simulink model "PathPlanningSample"  (R2019b)
settings: Solver=VariableStepAuto  StartTime=0.0  StopTime=10.0  RelTol=1e-3
settings Model: Creator=Mouleeswar  LastModifiedBy=naika

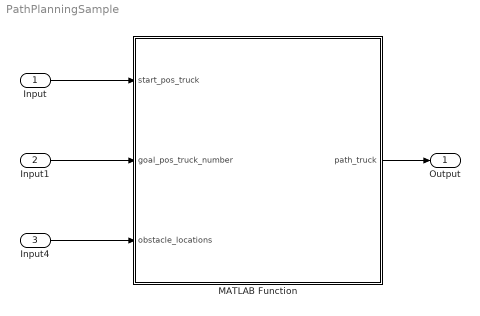
== system PathPlanningSample ==
  Input : Inport  OutDataTypeStr=double
  Input1 : Inport  Port=2  OutDataTypeStr=int16
  Input4 : Inport  Port=3  OutDataTypeStr=double
  MATLAB Function : MATLAB Function  TreatAsAtomicUnit=on
  Output : Outport  OutDataTypeStr=double
  wires:
  Input/1 -> MATLAB Function/1(start_pos_truck)
  Input1/1 -> MATLAB Function/2(goal_pos_truck_number)
  MATLAB Function/1(path_truck) -> Output/1
  Input4/1 -> MATLAB Function/3(obstacle_locations)

== matlab function PathPlanningSample/MATLAB Function ==
  data: start_pos_truck input; goal_pos_truck_number input; path_truck output; obstacle_locations input
function path_truck  = fcn(start_pos_truck, goal_pos_truck_number, obstacle_locations)
%% Input
S1 = start_pos_truck; %  [x-position y-position  angle  ]
E1 = goal_pos_truck_number; %  Dock number. Type:integer

obstacle = obstacle_locations; %Array containing the locations of all the obtacles. Example shown below.

%[ 5   6;
%  7   8;
% 100 500;
% 250 420;]

%% Output
%           [x-position y-position  angle   direction]
% units     [ meters      meters   radians      -    ]
% type      [ double      double    double   integer ]


% Ouput example
% path_truck1 = [100.01 100.02 1.56 1; % 
%                101.01 102.05 1.78 1;
%                101.01 102.05 1.78 -1;
%                101.01 102.05 1.78 -1];


    
edge = Map(obstacle);
costmap = vehicleCostmap(edge,'FreeThreshold',0.4);
 
vehicleDims = vehicleDimensions(98.5,19,'Wheelbase',62,'FrontOverhang',7.5,'RearOverhang',29);  % 4.5 m long, 1.7 m wide
NumCircles = 3;
ccConfig = inflationCollisionChecker(vehicleDims,'InflationRadius',5,'CenterPlacements',[0,0.5,1],'NumCircles',NumCircles);
costmap.CollisionChecker = ccConfig;

route = load('park_dock_points.mat')
routePlan = route.routePlan

dock_number = E1;
% park_number = 1;

% park = parking(park_number);
park = S1;
routePlan.StartPose(1,1) = park(1);
routePlan.StartPose(1,2) = park(2);
routePlan.StartPose(1,3) = park(3);


goal = docking(dock_number);
SP = HAS(goal,obstacle);

l=2;  % Number of wavepoints 

routePlan.EndPose(l,1) = SP(1);
routePlan.EndPose(l,2) = SP(2);
routePlan.EndPose(l,3) = SP(3);

routePlan.StartPose(l+1,1) = SP(1);
routePlan.StartPose(l+1,2) = SP(2);
routePlan.StartPose(l+1,3) = SP(3);
routePlan.EndPose(l+1,1) = goal(1);
routePlan.EndPose(l+1,2) = goal(2);
routePlan.EndPose(l+1,3) = goal(3);

% Striaght Path
routePlan.StartPose(l+2,1) = goal(1);
routePlan.StartPose(l+2,2) = goal(2);
routePlan.StartPose(l+2,3) = goal(3);
routePlan.EndPose(l+2,1) = goal(1);
routePlan.EndPose(l+2,2) = goal(2)+75;
routePlan.EndPose(l+2,3) = goal(3);        



figure(3)
plot(costmap)
hold on
helperPlotVehicle(routePlan{1, 'StartPose'}, vehicleDims, 'DisplayName', 'Current Pose')
legend

for i = 1:l+2
    if i <= l
        count =i
        currentPose = routePlan{i, 'StartPose'};
        goalPose = routePlan{i, 'EndPose'};
        motionPlanner = pathPlannerRRT(costmap,'MinTurningRadius',57,'MinIterations', 1000,'ApproximateSearch',false,'GoalBias',0.8,'GoalTolerance',[0.01,0.01,0.01],'ConnectionDistance', 5);
        refPath = plan(motionPlanner, currentPose, goalPose);
 
    else
        count =i
        currentPose = routePlan{i, 'StartPose'};
        goalPose = routePlan{i, 'EndPose'};
        motionPlanner = pathPlannerRRT(costmap,'MinTurningRadius',57,'MinIterations', 1000,'ConnectionMethod','Reeds-Shepp','ApproximateSearch',false,'GoalBias',0.8,'GoalTolerance',[0.01,0.01,0.01],'ConnectionDistance', 5);
        refPath = plan(motionPlanner, currentPose, goalPose);
    end
 
    [transitionPoses, directions] = interpolate(refPath);
    approxSeparation = 0.1; % meters
    numSmoothPoses   = round(refPath.Length / approxSeparation);
    [refPoses, directions, cumLengths, curvatures] = smoothPathSpline(transitionPoses, directions, numSmoothPoses);
    path_dir = [refPoses directions];
    if i==1
        final = path_dir;

    else
        final = cat(1,final,path_dir);
        
    end
    
end

for n = 1 : height(routePlan)
    
    vehiclePose = routePlan{n, 'EndPose'};
    legendEntry = sprintf('Goal %i', n);
    helperPlotVehicle(vehiclePose, vehicleDims, 'DisplayName', legendEntry);
    
end



hSmoothPath = plot(final(:, 1), final(:, 2), 'r', 'LineWidth', 2, ...
    'DisplayName', 'Smoothed Path');
hold off


path_truck = final;

end
